simulink model "AfferentTest"  (Simulink 8.4)
settings: Solver=ode45  StartTime=0.0  StopTime=10  RelTol=1e-3
libraries: NeuroModelerLibrary x1
settings Model: Creator=Bakhshiev  LastModifiedBy=Tim

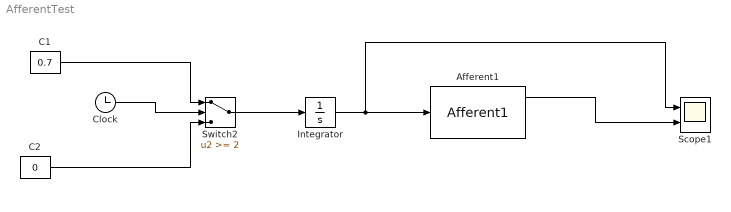
== system AfferentTest ==
  Afferent1 : NeuroModelerLibrary/Simple Cells/Afferent1  ExpCoeff=0.001  IncCoeff=0.999
  C1 : Constant  Value=0.7
  C2 : Constant  Value=0
  Clock : Clock
  Integrator : Integrator
  Scope1 : Scope  NumInputPorts=2
      settings: YMin=0~0  YMax=1~1  MaxDataPoints=500000
  Switch2 : Switch  Threshold=2  SaturateOnIntegerOverflow=on  InputSameDT=on
  wires:
  Clock/1 -> Switch2/2
  C2/1 -> Switch2/3
  C1/1 -> Switch2/1
  Switch2/1 -> Integrator/1
  Integrator/1 -> Afferent1/1, Scope1/1
  Afferent1/1 -> Scope1/2
